simulink model "ComputedTorque_DELTA"  (R2018b)
settings: Solver=FixedStepAuto  StartTime=0.0  StopTime=.5  FixedStep=0.001  RelTol=1e-5
model workspace (MAT data in the model file):
  I_bc = 0.466666666667
  I_bi = 2.46666666667
  I_brake = 1
  I_m = 1
  R = 0.63
  b = 2
  ee = [0; 0; -2.1944]
  k_r = 1
  l_A = 1
  l_B = 2
  m_b = 1
  m_br = 1.13333333333
  m_c = 0
  m_fb = 0.2
  m_n = 1
  m_nt = 3.6
  m_p = 0
  r_Gb = 0.558823529412
  r_l = 0.63
  r_m = 0.666666666667
  theta = [0 2.09439510239 4.18879020479]
values from neighbouring files (symbols this model uses):
  ddq_param_traj = [6*param_traj(1,:); 2*param_traj(2,:)]    [PtP_TrajGeneration.m]    (also in TrajGeneration.m)
  dq_param_traj = [3*param_traj(1,:); 2*param_traj(2,:); param_traj(3,:)]    [PtP_TrajGeneration.m]    (also in TrajGeneration.m)
  param_traj = nan(4,3)    [PtP_TrajGeneration.m]    (also in TrajGeneration.m; param_traj.mat = [0.59231523101  5.47421229733  2.21670604201; -1.92095980173)
  q_in = InvKin_DELTA(p_in)    [PtP_TrajGeneration.m]    (also in TrajGeneration.m)
settings Model: Creator=enrico  LastModifiedBy=enrico

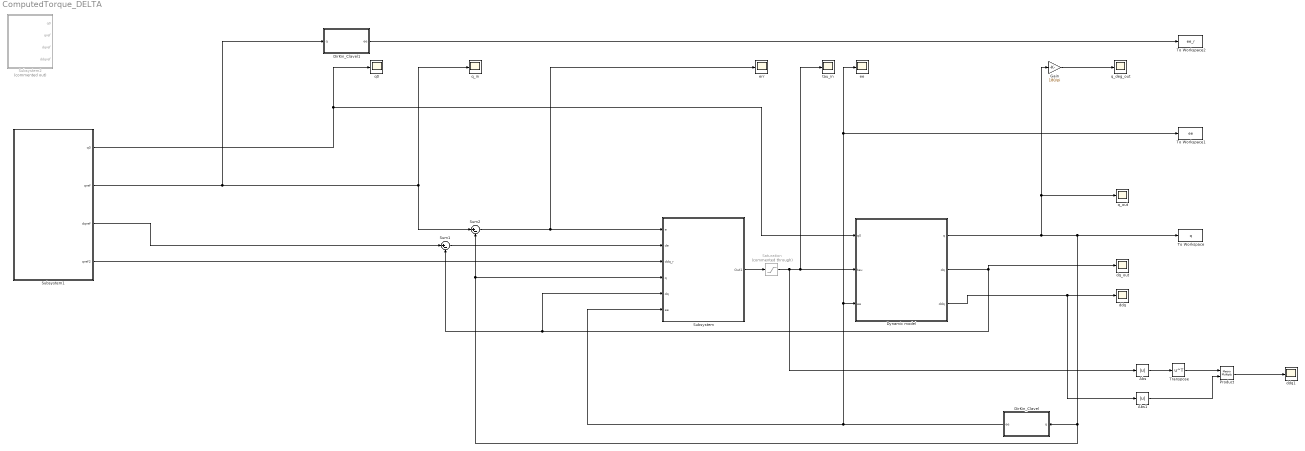
== system ComputedTorque_DELTA ==
  Abs : Abs
  Abs1 : Abs
  DirKin_Clavel : MATLAB Function  TreatAsAtomicUnit=on
      mask init:
      | loadvar
  DirKin_Clavel1 : MATLAB Function  TreatAsAtomicUnit=on
      mask init:
      | loadvar
  Dynamic model : Subsystem
  Gain : Gain  Gain=180/pi
  Product : Product  Multiplication=Matrix(*)
  Saturation : Saturate  Commented=through  UpperLimit=4000  LowerLimit=-4000  ZeroCross=off
  Subsystem : Subsystem  mask{K_p=100, K_d=20}
      mask prompts: K_p "Proportional_gain"; K_d "Derivative_gain"
  Subsystem1 : Subsystem
  Subsystem2 : Subsystem  Commented=on
  Sum1 : Sum  Inputs=|+-
  Sum2 : Sum  Inputs=|+-
  To Workspace : ToWorkspace  VariableName=q  SampleTime=-1
  To Workspace1 : ToWorkspace  VariableName=ee  SampleTime=-1
  To Workspace2 : ToWorkspace  VariableName=ee_r  SampleTime=-1
  Transpose : Math  Operator=transpose  SaturateOnIntegerOverflow=on
  ddq : Scope
  ddq1 : Scope
  "dq_out " : Scope
  "ee " : Scope
  err : Scope
  "q0 " : Scope
  "q_deg_out " : Scope
  q_in : Scope
  q_out : Scope
  tau_in : Scope
  wires:
  DirKin_Clavel/1(ee) -> Subsystem/6(ee), "ee "/1, To Workspace1/1, Dynamic model/3(ee)
  Gain/1 -> "q_deg_out "/1
  Dynamic model/3(ddq) -> Abs1/1, ddq/1
  Dynamic model/1(q) -> q_out/1, Gain/1, Subsystem/4(q), Sum2/2, DirKin_Clavel/1(q), To Workspace/1
  Subsystem1/2(qref) -> Sum2/1, q_in/1, DirKin_Clavel1/1(q)
  Subsystem1/1(q0) -> "q0 "/1, Dynamic model/1("q0 ")
  Sum2/1 -> Subsystem/1(e), err/1
  Dynamic model/2(dq) -> "dq_out "/1, Subsystem/5(dq), Sum1/2
  Subsystem/1(Out1) -> Saturation/1
  Sum1/1 -> Subsystem/2(de)
  Saturation/1 -> Abs/1, tau_in/1, Dynamic model/2(tau)
  Subsystem1/4(qref2) -> Subsystem/3(ddq_r)
  Subsystem1/3(dqref) -> Sum1/1
  DirKin_Clavel1/1(ee) -> To Workspace2/1
  Transpose/1 -> Product/1
  Abs/1 -> Transpose/1
  Abs1/1 -> Product/2
  Product/1 -> ddq1/1

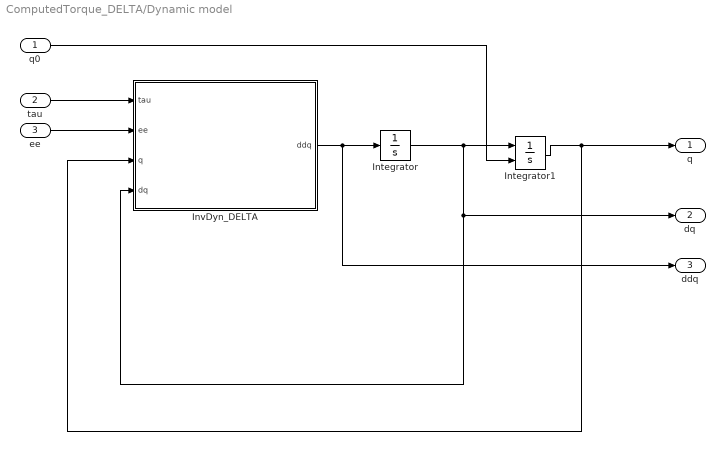
== system ComputedTorque_DELTA/Dynamic model ==
  "q0 " : Inport
  tau : Inport  Port=2
  ee : Inport  Port=3
  Integrator : Integrator  InitialCondition=[0; 0; 0]
  Integrator1 : Integrator  InitialConditionSource=external  InitialCondition=[pi/4; pi/4; pi/4]
  InvDyn_DELTA : MATLAB Function  TreatAsAtomicUnit=on
  q : Outport
  dq : Outport  Port=2
  ddq : Outport  Port=3
  wires:
  InvDyn_DELTA/1(ddq) -> ddq/1, Integrator/1
  ee/1 -> InvDyn_DELTA/2(ee)
  Integrator1/1 -> q/1, InvDyn_DELTA/3(q)
  Integrator/1 -> Integrator1/1, dq/1, InvDyn_DELTA/4(dq)
  tau/1 -> InvDyn_DELTA/1(tau)
  "q0 "/1 -> Integrator1/2

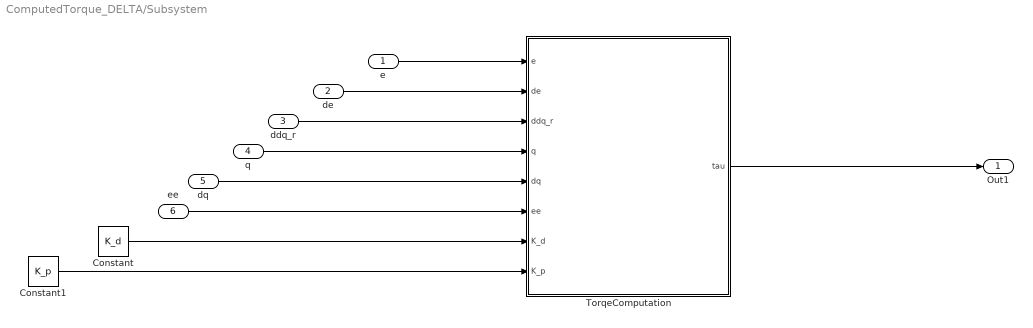
== system ComputedTorque_DELTA/Subsystem ==
  e : Inport
  de : Inport  Port=2
  ddq_r : Inport  Port=3
  q : Inport  Port=4
  dq : Inport  Port=5
  ee : Inport  Port=6
  Constant : Constant  Value=K_d
  Constant1 : Constant  Value=K_p
  TorqeComputation : MATLAB Function  TreatAsAtomicUnit=on
  Out1 : Outport
  wires:
  ddq_r/1 -> TorqeComputation/3(ddq_r)
  e/1 -> TorqeComputation/1(e)
  q/1 -> TorqeComputation/4(q)
  TorqeComputation/1(tau) -> Out1/1
  ee/1 -> TorqeComputation/6(ee)
  de/1 -> TorqeComputation/2(de)
  dq/1 -> TorqeComputation/5(dq)
  Constant/1 -> TorqeComputation/7(K_d)
  Constant1/1 -> TorqeComputation/8(K_p)

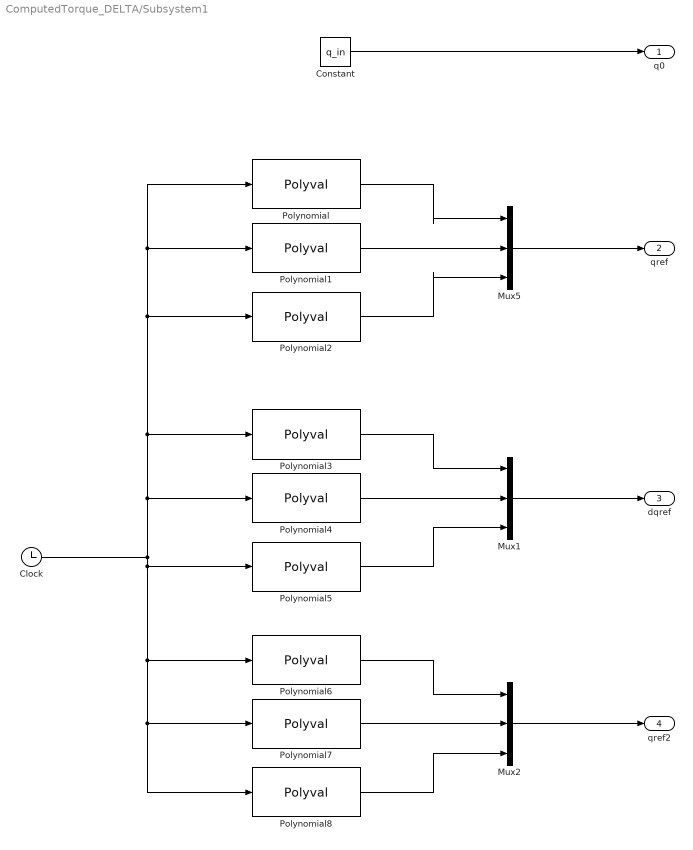
== system ComputedTorque_DELTA/Subsystem1 ==
  Clock : Clock
  Constant : Constant  Value=q_in
  Mux1 : Mux  Inputs=3
  Mux2 : Mux  Inputs=3
  Mux5 : Mux  Inputs=3
  Polynomial : Polyval  Coefs=param_traj(:,1)
  Polynomial1 : Polyval  Coefs=param_traj(:,2)
  Polynomial2 : Polyval  Coefs=param_traj(:,3)
  Polynomial3 : Polyval  Coefs=dq_param_traj(:,1)
  Polynomial4 : Polyval  Coefs=dq_param_traj(:,2)
  Polynomial5 : Polyval  Coefs=dq_param_traj(:,3)
  Polynomial6 : Polyval  Coefs=ddq_param_traj(:,1)
  Polynomial7 : Polyval  Coefs=ddq_param_traj(:,2)
  Polynomial8 : Polyval  Coefs=ddq_param_traj(:,3)
  q0 : Outport
  qref : Outport  Port=2
  dqref : Outport  Port=3
  qref2 : Outport  Port=4
  wires:
  Mux5/1 -> qref/1
  Polynomial/1 -> Mux5/1
  Polynomial1/1 -> Mux5/2
  Polynomial2/1 -> Mux5/3
  Polynomial5/1 -> Mux1/3
  Polynomial4/1 -> Mux1/2
  Polynomial3/1 -> Mux1/1
  Mux1/1 -> dqref/1
  Mux2/1 -> qref2/1
  Polynomial6/1 -> Mux2/1
  Polynomial7/1 -> Mux2/2
  Polynomial8/1 -> Mux2/3
  Clock/1 -> Polynomial4/1, Polynomial3/1, Polynomial2/1, Polynomial1/1, Polynomial/1, Polynomial8/1, Polynomial7/1, Polynomial6/1, Polynomial5/1
  Constant/1 -> q0/1

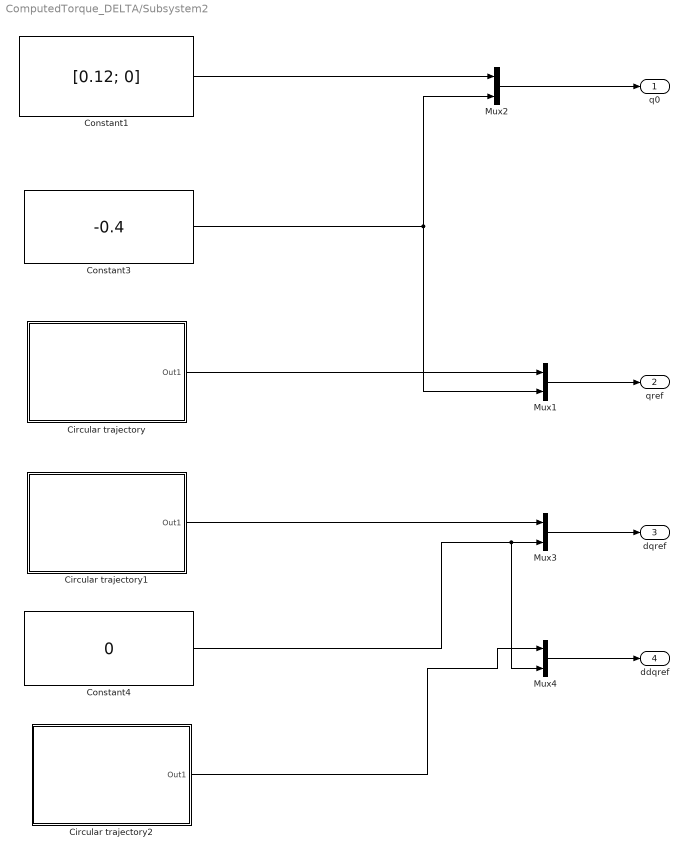
== system ComputedTorque_DELTA/Subsystem2 ==
  Circular trajectory : Subsystem  mask{A=0.12, F=3}
      mask prompts: A "Amplitude"; F "Frequency"
  Circular trajectory1 : Subsystem  mask{A=0.12, F=3}
      mask prompts: A "Amplitude"; F "Frequency"
  Circular trajectory2 : Subsystem  mask{A=0.12, F=3}
      mask prompts: A "Amplitude"; F "Frequency"
  Constant1 : Constant  Value=[0.12; 0]
  Constant3 : Constant  Value=-0.4
  Constant4 : Constant  Value=0
  Mux{1..4} (4 alike) : Mux  Inputs=2
  q0 : Outport
  qref : Outport  Port=2
  dqref : Outport  Port=3
  ddqref : Outport  Port=4
  wires:
  Mux4/1 -> ddqref/1
  Constant4/1 -> Mux3/2, Mux4/2
  Mux3/1 -> dqref/1
  Circular trajectory2/1(Out1) -> Mux4/1
  Mux2/1 -> q0/1
  Mux1/1 -> qref/1
  Circular trajectory/1(Out1) -> Mux1/1
  Circular trajectory1/1(Out1) -> Mux3/1
  Constant3/1 -> Mux2/2, Mux1/2
  Constant1/1 -> Mux2/1

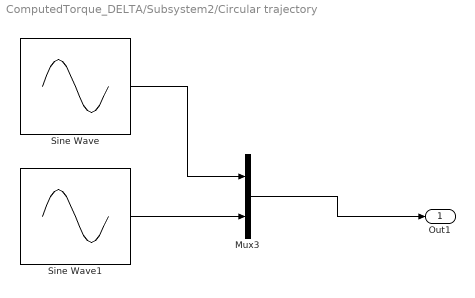
== system ComputedTorque_DELTA/Subsystem2/Circular trajectory ==
  Mux3 : Mux  Inputs=2
  Sine Wave : Sin  Amplitude=A  Frequency=F  Phase=pi/2  SampleTime=0
  Sine Wave1 : Sin  Amplitude=A  Frequency=F  SampleTime=0
  Out1 : Outport
  wires:
  Sine Wave1/1 -> Mux3/2
  Sine Wave/1 -> Mux3/1
  Mux3/1 -> Out1/1

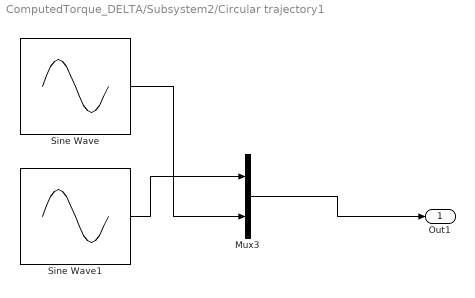
== system ComputedTorque_DELTA/Subsystem2/Circular trajectory1 ==
  Mux3 : Mux  Inputs=2
  Sine Wave : Sin  Amplitude=A  Frequency=F  Phase=pi/2  SampleTime=0
  Sine Wave1 : Sin  Amplitude=A  Frequency=F  SampleTime=0
  Out1 : Outport
  wires:
  Mux3/1 -> Out1/1
  Sine Wave/1 -> Mux3/2
  Sine Wave1/1 -> Mux3/1

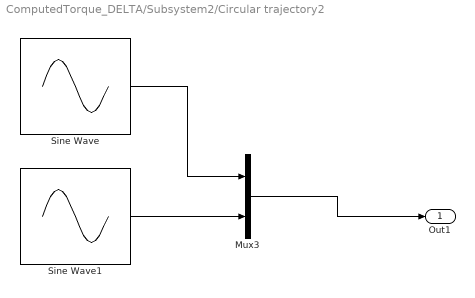
== system ComputedTorque_DELTA/Subsystem2/Circular trajectory2 ==
  Mux3 : Mux  Inputs=2
  Sine Wave : Sin  Amplitude=A  Frequency=F  Phase=pi/2  SampleTime=0
  Sine Wave1 : Sin  Amplitude=A  Frequency=F  SampleTime=0
  Out1 : Outport
  wires:
  Mux3/1 -> Out1/1
  Sine Wave/1 -> Mux3/1
  Sine Wave1/1 -> Mux3/2

== matlab function ComputedTorque_DELTA/DirKin_Clavel1 ==
  data: q input; ee output
function ee = DirKin_Clavel(q)

[theta, R, ~, ~, l_A, ~, ~, l_B, ~, ~, ~] = Parameters_DELTA;

D = nan(3,1);
E = nan(3,1);
F = nan(3,1);
G = nan(3,1);

for i = 1:3
   D(i) = -l_B^2 + l_A^2 + R^2 + 2*R*l_A*cos(q(i));
   
   E(i) = 2*(R + l_A*cos(q(i)))*cos(theta(i));
   
   F(i) = 2*(R + l_A*cos(q(i)))*sin(theta(i));
   
   G(i) = -2*l_A*sin(q(i)); 
end

H = [E(1)*G(2) - E(1)*G(3) - E(2)*G(1) + E(2)*G(3) + E(3)*G(1) - E(3)*G(2);
    -E(1)*F(2) + E(1)*F(3) + E(2)*F(1) - E(2)*F(3) - E(3)*F(1) + E(3)*F(2);
    -E(1)*D(2) + E(1)*D(3) + E(2)*D(1) - E(2)*D(3) - E(3)*D(1) + E(3)*D(2);
     F(1)*D(2) - F(1)*D(3) - F(2)*D(1) + F(2)*D(3) + F(3)*D(1) - F(3)*D(2);
    -F(1)*G(2) + F(1)*G(3) + F(2)*G(1) - F(2)*G(3) - F(3)*G(1) + F(3)*G(2)];

L = (H(5)^2 + H(1)^2)/H(2)^2 + 1;

M = 2*(H(5)*H(4) + H(1)*H(3))/H(2)^2 - (H(5)*E(1) + H(1)*F(1))/H(2) - G(1);

N = (H(4)^2 + H(3)^2)/H(2)^2 - (H(4)*E(1) + H(3)*F(1))/H(2) + D(1);

ee = nan(3,1);
ee2 = nan(3,1);

ee(3) = (-M + sqrt(M^2 - 4*L*N))/(2*L);

ee(1) = ee(3)*H(5)/H(2) + H(4)/H(2);

ee(2) = ee(3)*H(1)/H(2) + H(3)/H(2);

ee2(3) = (-M - sqrt(M^2 - 4*L*N))/(2*L);

ee2(1) = ee2(3)*H(5)/H(2) + H(4)/H(2);

ee2(2) = ee2(3)*H(1)/H(2) + H(3)/H(2);
 


% if ee2(3) < 0 
%     ee = ee2;
% end

if ee(3) > ee2(3)
    ee = ee2;
end

end

== matlab function ComputedTorque_DELTA/Dynamic model/InvDyn_DELTA ==
  data: tau input; ddq output; ee input; q input; dq input
function ddq = InvDyn_DELTA(tau, ee, q, dq)
% References:
% [1] Olsson, A. (2009). Modelling and control of a Delta-3 robot, (February).
% [2] Codourey, A. (1998). Dynamic Modeling of Parallel Robots for Computed-Torque Control Implementation, 17(12), 1325–1336.

% B, C, G matrices
[B, C, G, F] = BCG_DELTA(ee,q);


% Inverse dynamic
ddq = B\(tau - C*dq - G - F*dq); % Think adding friction coefficient of the manipulator (from [1] pg 27) 


end

== matlab function ComputedTorque_DELTA/DirKin_Clavel ==
  data: q input; ee output
function ee = DirKin_Clavel(q)

[theta, R, ~, ~, l_A, ~, ~, l_B, ~, ~, ~] = Parameters_DELTA;

D = nan(3,1);
E = nan(3,1);
F = nan(3,1);
G = nan(3,1);

for i = 1:3
   D(i) = -l_B^2 + l_A^2 + R^2 + 2*R*l_A*cos(q(i));
   
   E(i) = 2*(R + l_A*cos(q(i)))*cos(theta(i));
   
   F(i) = 2*(R + l_A*cos(q(i)))*sin(theta(i));
   
   G(i) = -2*l_A*sin(q(i)); 
end

H = [E(1)*G(2) - E(1)*G(3) - E(2)*G(1) + E(2)*G(3) + E(3)*G(1) - E(3)*G(2);
    -E(1)*F(2) + E(1)*F(3) + E(2)*F(1) - E(2)*F(3) - E(3)*F(1) + E(3)*F(2);
    -E(1)*D(2) + E(1)*D(3) + E(2)*D(1) - E(2)*D(3) - E(3)*D(1) + E(3)*D(2);
     F(1)*D(2) - F(1)*D(3) - F(2)*D(1) + F(2)*D(3) + F(3)*D(1) - F(3)*D(2);
    -F(1)*G(2) + F(1)*G(3) + F(2)*G(1) - F(2)*G(3) - F(3)*G(1) + F(3)*G(2)];

L = (H(5)^2 + H(1)^2)/H(2)^2 + 1;

M = 2*(H(5)*H(4) + H(1)*H(3))/H(2)^2 - (H(5)*E(1) + H(1)*F(1))/H(2) - G(1);

N = (H(4)^2 + H(3)^2)/H(2)^2 - (H(4)*E(1) + H(3)*F(1))/H(2) + D(1);

ee = nan(3,1);
ee2 = nan(3,1);

ee(3) = (-M + sqrt(M^2 - 4*L*N))/(2*L);

ee(1) = ee(3)*H(5)/H(2) + H(4)/H(2);

ee(2) = ee(3)*H(1)/H(2) + H(3)/H(2);

ee2(3) = (-M - sqrt(M^2 - 4*L*N))/(2*L);

ee2(1) = ee2(3)*H(5)/H(2) + H(4)/H(2);

ee2(2) = ee2(3)*H(1)/H(2) + H(3)/H(2);
 


% if ee2(3) < 0 
%     ee = ee2;
% end

if ee(3) > ee2(3)
    ee = ee2;
end

end

== matlab function ComputedTorque_DELTA/Subsystem/TorqeComputation ==
  data: e input; de input; ddq_r input; q input; tau output; dq input; ee input; K_d input; K_p input
function tau = fcn(e, de, ddq_r, q, dq, ee, K_d, K_p)

[B, C, G, F] = BCG_DELTA(ee,q);

tau = B*(ddq_r + K_d*de + K_p * e) + F*dq + C*dq + G;

end
